simulink model "GPI_Ball_Beam"  (R2014a)
settings: Solver=ode14x  SolverMode=SingleTasking  StartTime=0.0  StopTime=10.0  FixedStep=0.0001  RelTol=1e-3
undefined symbols (not defined in the file): k, k0, k1, k2, k3, k4, k5, k6, k7, wt, Xit
settings Model: CovMetricSettings=dwe  CovHtmlReporting=off  covSaveCumulativeToWorkspaceVar=off  CovSaveSingleToWorkspaceVar=off  CovExternalEMLEnable=on  CovSFcnEnable=on  Creator=cheng  LastModifiedBy=cheng
settings DataIOCC: LimitDataPoints=off  SaveFormat=StructureWithTime
settings DebuggingCC: MergeDetectMultiDrivingBlocksExec=error  SolverPrmCheckMsg=none  FrameProcessingCompatibilityMsg=error  SFUnexpectedBacktrackingDiag=error  SFNoUnconditionalDefaultTransitionDiag=error
settings HardwareCC: ProdBitPerPointer=64  ProdLargestAtomicFloat=Float  ProdIntDivRoundTo=Zero  ProdEndianess=LittleEndian  ProdHWDeviceType=Specified
settings ModelReferenceCC: PropagateSignalLabelsOutOfModel=on
settings SFSimCC: SimUseLocalCustomCode=on
settings RTWCC: RTWUseLocalCustomCode=on
settings GRTTargetCC: TargetLangStandard=C99 (ISO)  GeneratePreprocessorConditionals=Use local settings

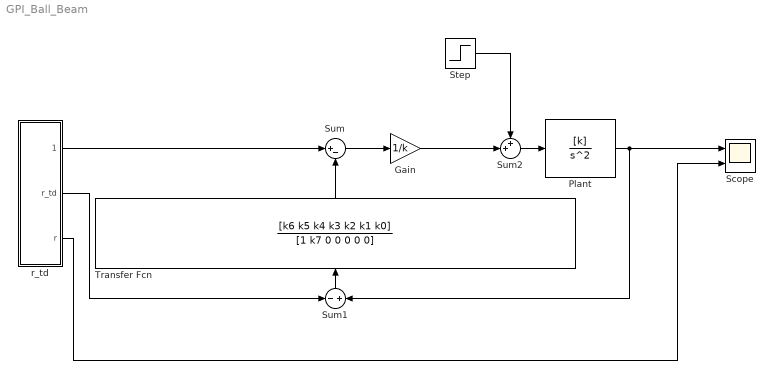
== system GPI_Ball_Beam ==
  Gain : Gain  Gain=1/k
  Plant : TransferFcn  Numerator=[k]  Denominator=[1 0 0]
  Scope : Scope  NumInputPorts=2
      settings: TimeRange=auto  MaxDataPoints=5000  SaveToWorkspace=off  SaveName=ScopeData  YMin=0.96434~-5  YMax=1.0337~5  SampleTime=-1
  Step : Step  Time=5  After=1000  SampleTime=0
  Sum : Sum  Inputs=|+-
  Sum1 : Sum  Inputs=-|+
  Sum2 : Sum  Inputs=++|
  Transfer Fcn : TransferFcn  Numerator=[k6 k5 k4 k3 k2 k1 k0]  Denominator=[1 k7 0 0 0 0 0]
  r_td : Subsystem
  wires:
  Plant/1 -> Sum1/2, Scope/1
  Gain/1 -> Sum2/2
  Sum/1 -> Gain/1
  Transfer Fcn/1 -> Sum/2
  Sum1/1 -> Transfer Fcn/1
  r_td/2(r_td) -> Sum1/1
  r_td/1(rdd_td) -> Sum/1
  Sum2/1 -> Plant/1
  Step/1 -> Sum2/1
  r_td/3(r) -> Scope/2

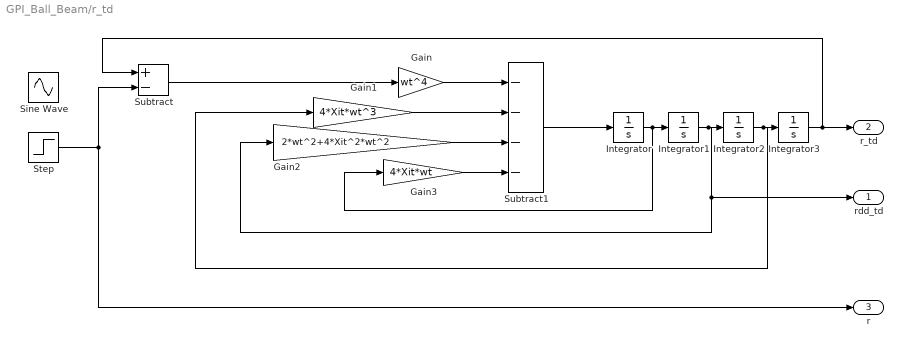
== system GPI_Ball_Beam/r_td ==
  Gain : Gain  Gain=wt^4
  Gain1 : Gain  Gain=4*Xit*wt^3
  Gain2 : Gain  Gain=2*wt^2+4*Xit^2*wt^2
  Gain3 : Gain  Gain=4*Xit*wt
  Integrator{,1..3} (4 alike) : Integrator
  Sine Wave : Sin  SampleTime=0
  Step : Step  SampleTime=0
  Subtract : Sum  Inputs=+-
  Subtract1 : Sum  Inputs=----
  rdd_td : Outport
  r_td : Outport  Port=2
  r : Outport  Port=3
  wires:
  Step/1 -> Subtract/2, r/1
  Integrator1/1 -> Gain2/1, rdd_td/1, Integrator2/1
  Integrator3/1 -> Subtract/1, r_td/1
  Integrator2/1 -> Gain1/1, Integrator3/1
  Integrator/1 -> Gain3/1, Integrator1/1
  Subtract/1 -> Gain/1
  Gain/1 -> Subtract1/1
  Gain1/1 -> Subtract1/2
  Gain2/1 -> Subtract1/3
  Gain3/1 -> Subtract1/4
  Subtract1/1 -> Integrator/1
